simulink model "Lab3_DigitalModulation"  (R2019b)
settings: Solver=FixedStepDiscrete  StartTime=0.0  StopTime=inf  FixedStep=1/fs  RelTol=1e-3
values from neighbouring files (symbols this model uses):
  binary = audioToBinary(wav, [bits_per_symbol])    [Lab3_DigitalModulation.m]    (also in audioToBinary.m = bin2dec(char_reshaped'))
undefined symbols (not defined in the file or in its folder): fs
libraries: commdigbbndam3 x2, commchan3 x1, commsink2 x1, impairlib x1, dspsrcs4 x1
settings Model: Creator=Emilija  LastModifiedBy=20182201

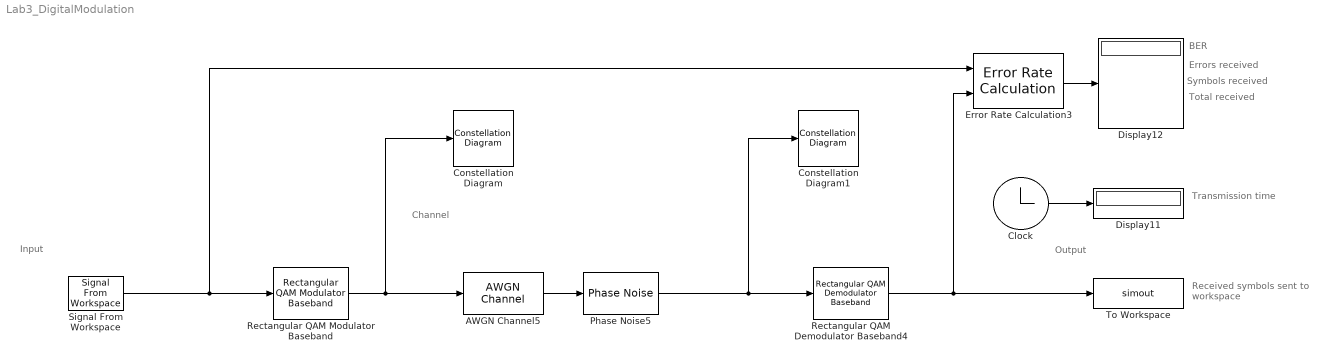
== system Lab3_DigitalModulation ==
  note: Output
  note: Errors received
  note: Symbols received
  note: BER
  note: Channel
  note: Transmission time
  note: Received symbols sent to workspace
  note: Input
  note: Total received
  AWGN Channel5 : commchan3/AWGN Channel  InputProcessing=Columns as channels (frame based)  seed=54321  noiseMode="Signal to noise ratio  (SNR)"  EbNodB=15  EsNodB=40  SNRdB=20  bitsPerSym=2  Ps=1  Tsym=1e-6  variance=1
      settings: SourceProductName=Communications Toolbox
  Clock : Clock
      settings: Decimation=1000
  Constellation Diagram : ConstellationDiagram
  Constellation Diagram1 : ConstellationDiagram
  Display11 : Display
      settings: Decimation=1000
  Display12 : Display
  Error Rate Calculation3 : commsink2/Error Rate Calculation  N=0  st_delay=0  cp_mode=Entire frame  subframe=[]  PMode=Port  WsName=ErrorVec  RsMode2=off  stop=on  numErr=inf  maxBits=length(binary)
      settings: SourceProductName=Communications Toolbox
  Phase Noise5 : impairlib/Phase Noise  Level=-70  FrequencyOffset=1000  SampleRate=1e3  RandomStream=mt19937ar with seed  Seed=2137  SimulateUsing=Interpreted execution
      settings: SourceProductName=SerDes Toolbox  SourceProductBaseCode=SX
  Rectangular QAM Demodulator Baseband4 : commdigbbndam3/Rectangular QAM Demodulator Baseband  M=16  OutType=Integer  DecType=Hard decision  VarSource=Dialog  Variance=1  Dec=Binary  Mapping=[0:15]  PowType=Average Power  MinDist=2  AvgPow=1  PeakPow=1  Ph=0  outDtype1=Inherit via internal rule  outDtype2=Inherit via internal rule  derotateFactorWordLen=16  derotateFactorDataTypeStr=Inherit: Same word length as input  derotateFactorLastDataTypeStr=Inherit: Same word length as input  denormFactorWordLen=16  denormFactorDataTypeStr=Inherit: Same word length as input  denormFactorLastDataTypeStr=Inherit: Same word length as input  prodOutWordLen=32  prodOutOverflowMode=Wrap  prodOutRoundingMode=Floor  prodOutOvFlMode=off  prodOutOvFlModeLastStrValue=off  sumWordLen=32
      settings: SourceProductName=Communications Toolbox
  Rectangular QAM Modulator Baseband : commdigbbndam3/Rectangular QAM Modulator Baseband  M=16  InType=Integer  Enc=Binary  Mapping=[0:15]  PowType=Average Power  MinDist=2  AvgPow=1  PeakPow=1  Ph=0  outDtype=double  outWordLen=16  outUDDataType=sfix(16)  outFracLenMode=Best precision  outFracLen=15  outDataTypeStr=double  outLastDataTypeStr=double
      settings: SourceProductName=Communications Toolbox
  Signal From Workspace : dspsrcs4/Signal From Workspace  X=binary  Ts=1/fs  nsamps=1  OutputAfterFinalValue=Cyclic repetition  ignoreOrWarnInputAndFrameLengths=off  OutputFrames=off
  To Workspace : ToWorkspace  VariableName=simout  SampleTime=-1
      settings: Save2DSignal=2-D array (concatenate along first dimension)
  wires:
  Clock/1 -> Display11/1
  Rectangular QAM Demodulator Baseband4/1 -> Error Rate Calculation3/2, To Workspace/1
  Error Rate Calculation3/1 -> Display12/1
  AWGN Channel5/1 -> Phase Noise5/1
  Phase Noise5/1 -> Rectangular QAM Demodulator Baseband4/1, Constellation Diagram1/1
  Signal From Workspace/1 -> Error Rate Calculation3/1, Rectangular QAM Modulator Baseband/1
  Rectangular QAM Modulator Baseband/1 -> AWGN Channel5/1, Constellation Diagram/1
